simulink model "VehicleModel_AdaptiveAutosar"  (R2022a)
settings: Solver=FixedStepDiscrete  StartTime=0.0  StopTime=10.0  RelTol=1e-3
model workspace (MATLAB code in the model file):
  | cmdLim = Simulink.Parameter;
  | cmdLim.Value = 15;
  | cmdLim.Description = 'Limit for controlling the maximum surface command angle.';
  | cmdLim.Min = 0;
  | cmdLim.Max = 90;
  | cmdLim.DocUnits = 'deg';
  | 
  | dispGain = Simulink.Parameter;
  | dispGain.Value = 0.75;
  | dispGain.Description = 'Gain applied to the displacement error.';
  | dispGain.Min = 0;
  | dispGain.Max = [];
  | dispGain.DocUnits = 'deg/sec/deg';
  | 
  | dispLim = Simulink.Parameter;
  | dispLim.Value = 30;
  | dispLim.Description = 'Limit for controlling the maximum commanded angle.';
  | dispLim.Min = 0;
  | dispLim.Max = 180;
  | dispLim.DocUnits = 'deg';
  | 
  | intGain = Simulink.Parameter;
  | intGain.Value = 0.5;
  | intGain.Description = 'Gain applied to the integral error.';
  | intGain.Min = 0;
  | intGain.Max = [];
  | intGain.DocUnits = 'deg/sec/deg/sec';
  | 
  | intLim = Simulink.Parameter;
  | intLim.Value = 5;
  | intLim.Description = 'Limit for controlling the maximum commanded angle.';
  | intLim.Min = 0;
  | intLim.Max = 90;
  | intLim.DocUnits = 'deg';
  | 
  | rateGain = Simulink.Parameter;
  | rateGain.Value = 2;
  | rateGain.Description = 'Gain applied to the rate error.';
  | rateGain.Min = 0;
  | rateGain.Max = [];
  | rateGain.DocUnits = 'deg/deg/sec';
  | 
  | rateLim = Simulink.Parameter;
  | rateLim.Value = 6;
  | rateLim.Description = 'Limit for controlling the maximum commanded angle.';
  | rateLim.Min = 0;
  | rateLim.Max = 180;
  | rateLim.DocUnits = 'deg/sec';
  | 
  | hdgGain = Simulink.Parameter;
  | hdgGain.Value = 0.015;
values from neighbouring files (symbols this model uses):
  DRIVER_EYES_OFF = Simulink.Parameter    [InitialValueFile.m]
  DRIVER_EYES_ON = Simulink.Parameter    [InitialValueFile.m]
  DRIVER_READINESS_HIGH = Simulink.Parameter    [InitialValueFile.m]
  DRIVER_READINESS_MEDIUM = Simulink.Parameter    [InitialValueFile.m]
  DRIVER_SEATED_ON = Simulink.Parameter    [InitialValueFile.m]
libraries: autosarlibaprouting x9, simulink x6
settings Model: RequirementInfo={} %GIDa_fe9045fd_0412_4b6e_8206_617cc20e6fde  FPTRunName=Active  Creator=HP  LastModifiedBy=HP
settings SolverCC: ConcurrentTasks=on  AlgebraicLoopSolver=TrustRegion  InsertRTBMode=Never (minimum delay)  MaxZcPerStep=1
settings DataIOCC: SaveOutput=off  SignalLogging=off  DSMLogging=off  SaveTime=off
settings OptimizationCC: DefaultParameterBehavior=Inlined  UseFloatMulNetSlope=on  UseSpecifiedMinMax=on  InlineInvariantSignals=on  EnhancedBackFolding=on  PassReuseOutputArgsAs=Individual arguments  ZeroExternalMemoryAtStartup=off  ZeroInternalMemoryAtStartup=off  NoFixptDivByZeroProtection=on  EfficientFloat2IntCast=on  OptimizeBlockOrder=speed  DifferentSizesBufferReuse=on  OptimizationCustomize=off  EfficientTunableParamExpr=on
settings DebuggingCC: ParameterTunabilityLossMsg=error  UnconnectedInputMsg=warning  UnconnectedOutputMsg=warning  UnconnectedLineMsg=warning  SFUnexpectedBacktrackingDiag=warning  SFNoUnconditionalDefaultTransitionDiag=warning  SFExecutionAtInitializationDiag=none  SFMachineParentedDataDiag=warning  ArithmeticOperatorsInVariantConditions=warning
settings HardwareCC: ProdLongLongMode=on
settings SFSimCC: SimGenImportedTypeDefs=on  MATLABDynamicMemAlloc=off  SimTargetLang=C++
settings RTWCC: Description=AUTOSAR Adaptive  SystemTargetFile=autosar_adaptive.tlc  GenCodeOnly=on  TemplateMakefile=ert_default_tmf  Toolchain=AUTOSAR Adaptive | CMake  BuildConfiguration=Faster Runs  IncludeHyperlinkInReport=on  TargetLang=C++  DLArmComputeVersion=19.05
settings CodeAppCC: ForceParamTrailComments=on  IgnoreCustomStorageClasses=off  MaxIdLength=63  OperatorAnnotations=on  SimulinkDataObjDesc=on  SFDataObjDesc=on  CustomSymbolStrGlobalVar=rt$N$M  CustomSymbolStrType=$N$M  CustomSymbolStrFcn=$N$M$F  CustomSymbolStrMacro=$N$M  InsertBlockDesc=on  EnableCustomComments=on  ReqsInCode=on
settings AUTOSARAdaptiveTargetCC: TargetFcnLib=ansi_tfl_table_tmw.mat  GenFloatMathFcnCalls=NOT IN USE  TargetLangStandard=C++11 (ISO)  CodeReplacementLibrary=None  UtilityFuncGeneration=Auto  MultiwordTypeDef=System defined  MultiwordLength=2048  DynamicStringBufferSize=256  GenerateFullHeader=on  InferredTypesCompatibility=off  GenerateSampleERTMain=off  GenerateTestInterfaces=off  ModelReferenceCompliant=on  ParMdlRefBuildCompliant=on  CompOptLevelCompliant=on  ConcurrentExecutionCompliant=on  IncludeMdlTerminateFcn=on  CombineOutputUpdateFcns=on  CombineSignalStateStructs=off  GroupInternalDataByFunction=off  SuppressErrorStatus=on  IncludeFileDelimiter=Auto  ERTCustomFileBanners=off  SupportAbsoluteTime=on  LogVarNameModifier=rt_  MatFileLogging=off  CodeInterfacePackaging=C++ class  PurelyIntegerCode=off  SupportNonFinite=off  SupportComplex=on  SupportContinuousTime=off  SupportNonInlinedSFcns=off  RemoveDisableFunc=off  RemoveResetFunc=on  SupportVariableSizeSignals=off  ParenthesesLevel=Nominal  CastingMode=Nominal  MATLABClassNameForMDSCustomization=Simulink.SoftwareTarget.TargetSpecificTriggerConfigurationBase  ModelStepFunctionPrototypeControlCompliant=off  CPPClassGenCompliant=on  AutosarCompliant=on  MDXCompliant=off  GRTInterface=off  GenerateAllocFcn=off  UseToolchainInfoCompliant=on  GenerateSharedConstants=on  CoderGroups=[]  AccessMethods=[]  LookupTableObjectStructAxisOrder=2,1,3,4,...  LUTObjectStructOrderExplicitValues=Size,Breakpoints,Table  LUTObjectStructOrderEvenSpacing=Size,Table,Breakpoints  ArrayLayout=Column-major  UnsupportedSFcnMsg=error  ERTHeaderFileRootName=$R$E  ERTSourceFileRootName=$R$E  ERTDataFileRootName=$R_data  OptimizeReductions=off  GenerateASAP2=off  DSAsUniqueAccess=off  ExtMode=off  ExtModeTransport=0  ExtModeStaticAlloc=off  ExtModeStaticAllocSize=1000000  ExtModeTesting=off  ExtModeMexFile=ext_comm  UserDataClassName=[]  ExtModeIntrfLevel=Level1  InlinedParameterPlacement=NonHierarchical  TargetOS=BareBoardExample  MultiInstanceErrorCode=Error  RootIOFormat=Structure reference  RTWCAPISignals=off  RTWCAPIParams=off  RTWCAPIStates=off  RTWCAPIRootIO=off  ERTSrcFileBannerTemplate=ert_code_template.cgt  ERTHdrFileBannerTemplate=ert_code_template.cgt  ERTDataSrcFileTemplate=ert_code_template.cgt  ERTDataHdrFileTemplate=ert_code_template.cgt  ERTCustomFileTemplate=example_file_process.tlc  EnableDataOwnership=off  SignalDisplayLevel=10  ParamTuneLevel=10  GlobalDataDefinition=Auto  DataDefinitionFile=global.c  GlobalDataReference=Auto  ERTFilePackagingFormat=Modular  RateTransitionBlockCode=Inline  DataReferenceFile=global.h  PreserveExpressionOrder=off  PreserveIfCondition=off  ConvertIfToSwitch=on  PreserveExternInFcnDecls=on  PreserveStaticInFcnDecls=on  SuppressUnreachableDefaultCases=on  EnableSignedLeftShifts=on  EnableSignedRightShifts=on  ImplementImageWithCVMat=off  IndentStyle=K&R  IndentSize=2  NewlineStyle=Default  MaxLineWidth=80  EnableUserReplacementTypes=off  MaxIdInt64=MAX_int64_T  MinIdInt64=MIN_int64_T  MaxIdUint64=MAX_uint64_T  MaxIdInt32=MAX_int32_T  MinIdInt32=MIN_int32_T  MaxIdUint32=MAX_uint32_T  MaxIdInt16=MAX_int16_T  MinIdInt16=MIN_int16_T  MaxIdUint16=MAX_uint16_T  MaxIdInt8=MAX_int8_T  MinIdInt8=MIN_int8_T  MaxIdUint8=MAX_uint8_T  BooleanTrueId=true  BooleanFalseId=false  MemSecPackage=--- None ---  MemSecDataConstants=Default  MemSecDataIO=Default  MemSecDataInternal=Default  MemSecDataParameters=Default  MemSecFuncInitTerm=Default  MemSecFuncExecute=Default  MemSecFuncSharedUtil=Default  GroupConstants=Default  GroupRootInputs=Default  GroupRootOutputs=Default  GroupInternal=Default  GroupParameters=Default  GroupDataTransfer=Default  GroupSharedLocalDataStores=Default  GroupInstanceSpecificParameters=Default  GroupModelData=Default  ArrayContainerType=std::array  AutosarSchemaVersion=00048  AutosarMaxShortNameLength=128  AdaptiveAutosarXCPSlaveTransportLayer=None  AdaptiveAutosarXCPSlaveTCPIPAddress=127.0.0.1  AdaptiveAutosarXCPSlavePort=17725  AdaptiveAutosarXCPSlaveVerbosity=off  AdaptiveAutosarUseCustomXCPSlave=off
settings ConfigComp: CovScope=ReferencedModels  CovSaveName=covdata_rollAP  CovMetricSettings=dcmtrwe  CovHTMLOptions=-sRT=1 -aTS=1 -bRG=1 -bTC=1 -hTR=1 -nFC=0 -scm=1 -bcm=1 -xEv=0  CovSaveCumulativeToWorkspaceVar=on  CovSaveSingleToWorkspaceVar=on  CovCumulativeVarName=covCumulativeData_rollAP  CovReportOnPause=off  CovExternalEMLEnable=off  CovSFcnEnable=off

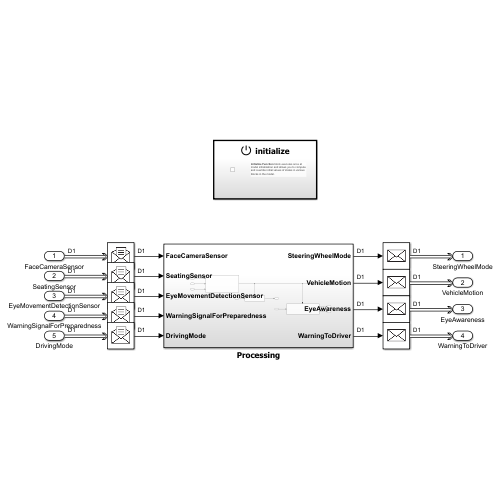
[thumbnail: Simulink's stored preview of the top-level diagram]
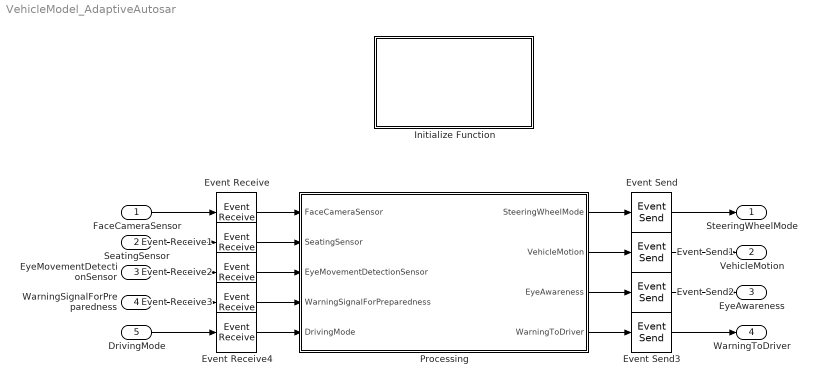
== system VehicleModel_AdaptiveAutosar ==
  FaceCameraSensor : Inport  OutputPortMessageModes=m
  SeatingSensor : Inport  OutputPortMessageModes=m  Port=2
  EyeMovementDetectionSensor : Inport  OutputPortMessageModes=m  Port=3
  WarningSignalForPreparedness : Inport  OutputPortMessageModes=m  Port=4
  DrivingMode : Inport  OutputPortMessageModes=m  Port=5
  Event Receive{,1..4} (5 alike) : autosarlibaprouting/Event Receive
      settings: SourceProductBaseCode=AS
  Event Send{,1..3} (4 alike) : autosarlibaprouting/Event Send
      settings: SourceProductBaseCode=AS
  Initialize Function : Subsystem  TreatAsAtomicUnit=on
  Processing : Subsystem  SystemSampleTime=1
  SteeringWheelMode : Outport  InputPortMessageModes=m  VectorParamsAs1DForOutWhenUnconnected=off
  VehicleMotion : Outport  InputPortMessageModes=m  Port=2  VectorParamsAs1DForOutWhenUnconnected=off
  EyeAwareness : Outport  InputPortMessageModes=m  Port=3  VectorParamsAs1DForOutWhenUnconnected=off
  WarningToDriver : Outport  InputPortMessageModes=m  Port=4  VectorParamsAs1DForOutWhenUnconnected=off
  wires:
  Event Receive/1 -> Processing/1(FaceCameraSensor)
  FaceCameraSensor/1 -> Event Receive/1
  Event Receive1/1 -> Processing/2(SeatingSensor)
  SeatingSensor/1 -> Event Receive1/1
  Event Receive2/1 -> Processing/3(EyeMovementDetectionSensor)
  EyeMovementDetectionSensor/1 -> Event Receive2/1
  Event Receive3/1 -> Processing/4(WarningSignalForPreparedness)
  WarningSignalForPreparedness/1 -> Event Receive3/1
  Event Receive4/1 -> Processing/5(DrivingMode)
  DrivingMode/1 -> Event Receive4/1
  Processing/1(SteeringWheelMode) -> Event Send/1
  Event Send/1 -> SteeringWheelMode/1
  Processing/2(VehicleMotion) -> Event Send1/1
  Event Send1/1 -> VehicleMotion/1
  Processing/3(EyeAwareness) -> Event Send2/1
  Event Send2/1 -> EyeAwareness/1
  Processing/4(WarningToDriver) -> Event Send3/1
  Event Send3/1 -> WarningToDriver/1

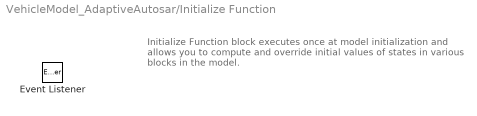
== system VehicleModel_AdaptiveAutosar/Initialize Function ==
  note: Initialize Function block executes once at model initialization and allows you to compute and override initial values of states in various blocks in the model.
  Event Listener : EventListener  DisableCoverage=on  EventName=reset

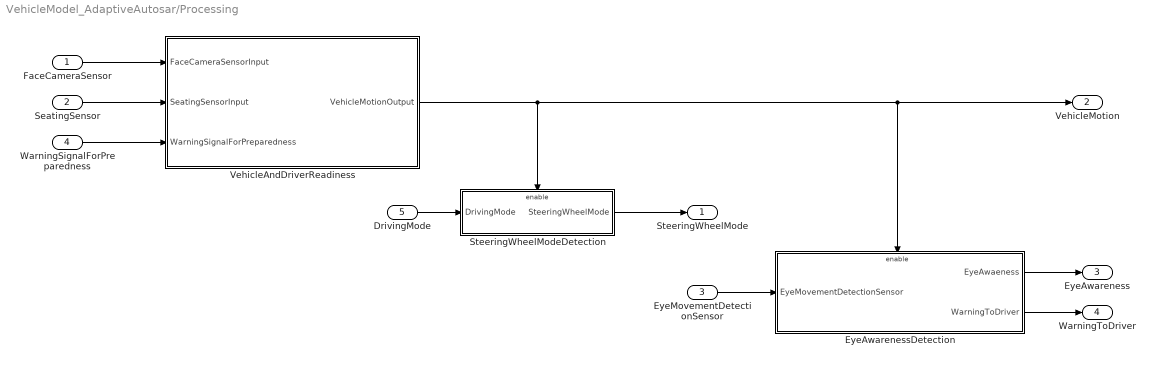
== system VehicleModel_AdaptiveAutosar/Processing ==
  FaceCameraSensor : Inport
  SeatingSensor : Inport  Port=2
  EyeMovementDetectionSensor : Inport  Port=3
  WarningSignalForPreparedness : Inport  Port=4
  DrivingMode : Inport  Port=5
  EyeAwarenessDetection : Subsystem
  SteeringWheelModeDetection : Subsystem
  VehicleAndDriverReadiness : Subsystem
  SteeringWheelMode : Outport  VectorParamsAs1DForOutWhenUnconnected=off
  VehicleMotion : Outport  Port=2  VectorParamsAs1DForOutWhenUnconnected=off
  EyeAwareness : Outport  Port=3
  WarningToDriver : Outport  Port=4
  wires:
  FaceCameraSensor/1 -> VehicleAndDriverReadiness/1(FaceCameraSensorInput)
  SeatingSensor/1 -> VehicleAndDriverReadiness/2(SeatingSensorInput)
  WarningSignalForPreparedness/1 -> VehicleAndDriverReadiness/3(WarningSignalForPreparedness)
  VehicleAndDriverReadiness/1(VehicleMotionOutput) -> VehicleMotion/1, EyeAwarenessDetection/Enable, SteeringWheelModeDetection/Enable
  EyeMovementDetectionSensor/1 -> EyeAwarenessDetection/1(EyeMovementDetectionSensor)
  SteeringWheelModeDetection/1(SteeringWheelMode) -> SteeringWheelMode/1
  EyeAwarenessDetection/1(EyeAwaeness) -> EyeAwareness/1
  DrivingMode/1 -> SteeringWheelModeDetection/1(DrivingMode)
  EyeAwarenessDetection/2(WarningToDriver) -> WarningToDriver/1

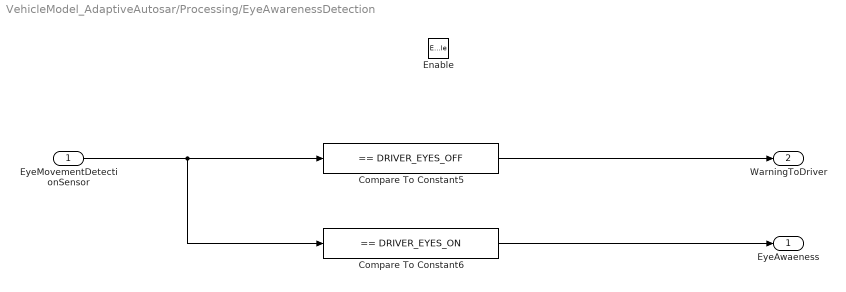
== system VehicleModel_AdaptiveAutosar/Processing/EyeAwarenessDetection ==
  EyeMovementDetectionSensor : Inport
  Enable : EnablePort
  Compare To Constant5 : simulink/Logic and Bit Operations/Compare To Constant  relop===  const=DRIVER_EYES_OFF  OutDataTypeStr=boolean
  Compare To Constant6 : simulink/Logic and Bit Operations/Compare To Constant  relop===  const=DRIVER_EYES_ON  OutDataTypeStr=boolean
  EyeAwaeness : Outport
  WarningToDriver : Outport  Port=2
  wires:
  Compare To Constant5/1 -> WarningToDriver/1
  Compare To Constant6/1 -> EyeAwaeness/1
  EyeMovementDetectionSensor/1 -> Compare To Constant6/1, Compare To Constant5/1

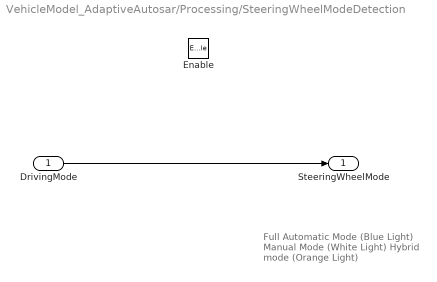
== system VehicleModel_AdaptiveAutosar/Processing/SteeringWheelModeDetection ==
  note: Full Automatic Mode (Blue Light)
      | Manual Mode (White Light)
      | Hybrid mode (Orange Light)
  DrivingMode : Inport
  Enable : EnablePort
  SteeringWheelMode : Outport
  wires:
  DrivingMode/1 -> SteeringWheelMode/1

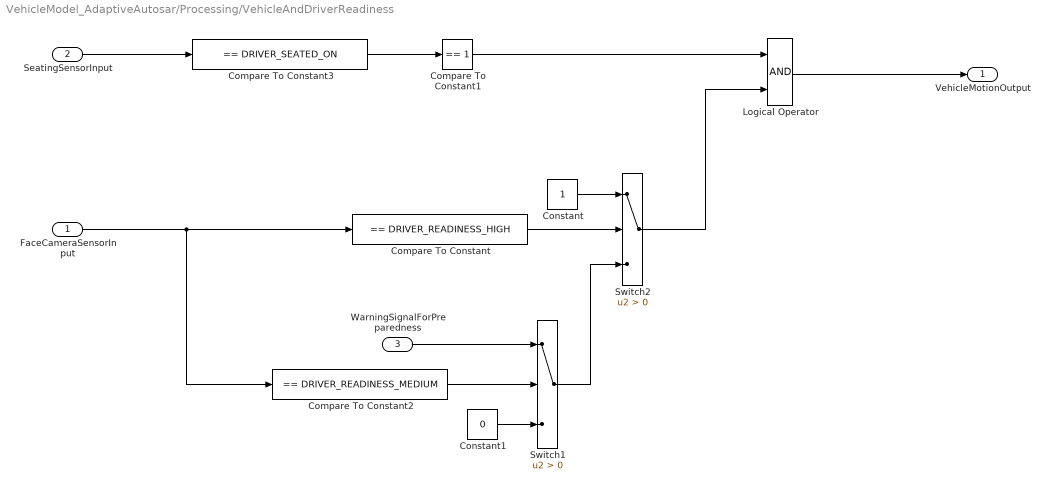
== system VehicleModel_AdaptiveAutosar/Processing/VehicleAndDriverReadiness ==
  FaceCameraSensorInput : Inport
  SeatingSensorInput : Inport  Port=2
  WarningSignalForPreparedness : Inport  Port=3
  Compare To Constant : simulink/Logic and Bit Operations/Compare To Constant  relop===  const=DRIVER_READINESS_HIGH  OutDataTypeStr=boolean
  Compare To Constant1 : simulink/Logic and Bit Operations/Compare To Constant  relop===  const=1  OutDataTypeStr=boolean
  Compare To Constant2 : simulink/Logic and Bit Operations/Compare To Constant  relop===  const=DRIVER_READINESS_MEDIUM  OutDataTypeStr=boolean
  Compare To Constant3 : simulink/Logic and Bit Operations/Compare To Constant  relop===  const=DRIVER_SEATED_ON  OutDataTypeStr=boolean
  Constant : Constant
  Constant1 : Constant  Value=0
  Logical Operator : Logic  AllPortsSameDT=off  OutDataTypeStr=boolean
  Switch1 : Switch  Criteria=u2 > Threshold  SaturateOnIntegerOverflow=off  InputSameDT=off
  Switch2 : Switch  Criteria=u2 > Threshold  SaturateOnIntegerOverflow=off  InputSameDT=off
  VehicleMotionOutput : Outport  VectorParamsAs1DForOutWhenUnconnected=off
  wires:
  Compare To Constant1/1 -> Logical Operator/1
  Switch1/1 -> Switch2/3
  Compare To Constant2/1 -> Switch1/2
  WarningSignalForPreparedness/1 -> Switch1/1
  Compare To Constant3/1 -> Compare To Constant1/1
  Compare To Constant/1 -> Switch2/2
  Constant/1 -> Switch2/1
  FaceCameraSensorInput/1 -> Compare To Constant/1, Compare To Constant2/1
  Constant1/1 -> Switch1/3
  SeatingSensorInput/1 -> Compare To Constant3/1
  Logical Operator/1 -> VehicleMotionOutput/1
  Switch2/1 -> Logical Operator/2
